simulink model "gftf"  (R2017b)
settings: Solver=VariableStepAuto  StartTime=0.0  StopTime=2  RelTol=1e-3
libraries: instrumentlib x2
settings Model: Creator=Administrador  LastModifiedBy=Administrador

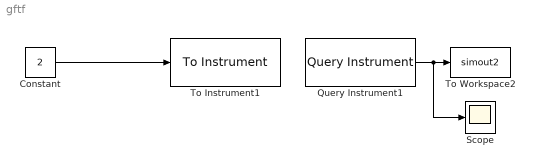
== system gftf ==
  Constant : Constant  Value=2
  Query Instrument1 : instrumentlib/Query Instrument  sampleTime=0.01  isWorkspaceObject=off  timeout=10  inputBufferSize=256  protocol=Serial  serialPort=COM1  baudRate=9600  gpibVendor=Agilent Technologies  boardIndex=0  primaryAddress=1  secondaryAddress=0  visaVendor=Agilent  visaSerialPort=0  chassisIndex=0  logicalAddress=0  tcpRemoteHost='127.0.0.1'  tcpRemotePort=4500  udpRemoteHost='127.0.0.1'  udpRemotePort=9090  visaTCPBoardIndex=0  visaTCPRemoteHost='127.0.0.1'  usbBoardIndex=0  usbManufID=0  usbModelCode=0  usbSerialNumber=0  initAction=None  initCommand='DATA:SOURCE CH1'  initFunction=get  queryCommand='curve?'  responseFormat=ASCII  asciiFormatting='%f'  precision=8-bit integer  byteOrder=Little endian  valuesToRead=1  removeBytes=off  afterOutputAction=Repeat query for new data  enableFrames=off  frameSize=1
      settings: SourceProductName=Instrument Control Toolbox  SourceProductBaseCode=IC
  Scope : Scope
  To Instrument1 : instrumentlib/To Instrument  sampleTime=0.01  isWorkspaceObject=off  timeout=10  inputBufferSize=256  protocol=Serial  serialPort=COM1  baudRate=9600  gpibVendor=Agilent Technologies  boardIndex=0  primaryAddress=1  secondaryAddress=0  visaVendor=Agilent  visaSerialPort=0  chassisIndex=0  logicalAddress=0  tcpRemoteHost='127.0.0.1'  tcpRemotePort=4500  udpRemoteHost='127.0.0.1'  udpRemotePort=9090  visaTCPBoardIndex=0  visaTCPRemoteHost='127.0.0.1'  usbBoardIndex=0  usbManufID=0  usbModelCode=0  usbSerialNumber=0  initAction=None  initCommand='DATA:SOURCE CH1'  initFunction=get  command=''  sendFormat=ASCII  asciiFormatting='%f'  precision=8-bit integer  byteOrder=Little endian
      settings: SourceProductName=Instrument Control Toolbox  SourceProductBaseCode=IC
  To Workspace2 : ToWorkspace  VariableName=simout2  SaveFormat=Timeseries  SampleTime=-1
  wires:
  Constant/1 -> To Instrument1/1
  Query Instrument1/1 -> Scope/1, To Workspace2/1
